simulink model "demo"  (R2019a)
settings: Solver=FixedStepAuto  StartTime=0.0  StopTime=inf  FixedStep=1  RelTol=1e-3
settings Model: Creator=Administrator  LastModifiedBy=Administrator

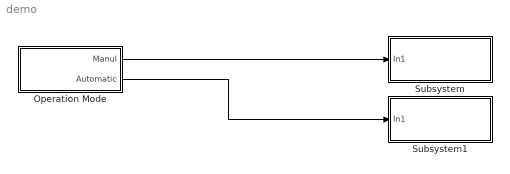
== system demo ==
  Operation Mode : Subsystem
  Subsystem : Subsystem
  Subsystem1 : Subsystem
  wires:
  Operation Mode/2(Automatic) -> Subsystem1/1(In1)
  Operation Mode/1("Manul ") -> Subsystem/1(In1)

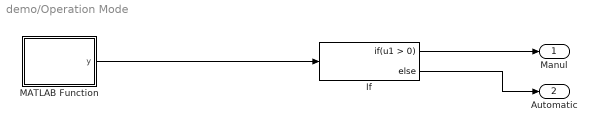
== system demo/Operation Mode ==
  If : If
  MATLAB Function : MATLAB Function  TreatAsAtomicUnit=on
  "Manul " : Outport
  Automatic : Outport  Port=2
  wires:
  If/1 -> "Manul "/1
  If/2 -> Automatic/1
  MATLAB Function/1(y) -> If/1

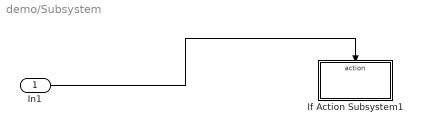
== system demo/Subsystem ==
  In1 : Inport
  If Action Subsystem1 : Subsystem  TreatAsAtomicUnit=on
  wires:
  In1/1 -> If Action Subsystem1/Action

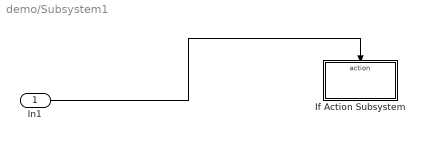
== system demo/Subsystem1 ==
  In1 : Inport
  If Action Subsystem : Subsystem  TreatAsAtomicUnit=on
  wires:
  In1/1 -> If Action Subsystem/Action

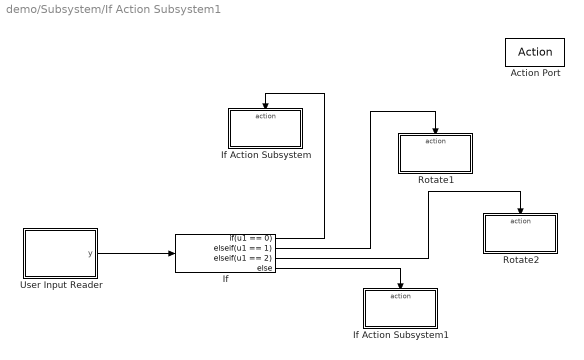
== system demo/Subsystem/If Action Subsystem1 ==
  Action Port : ActionPort
  If : If  IfExpression=u1 == 0  ElseIfExpressions=u1 == 1, u1 == 2
  If Action Subsystem : Subsystem  TreatAsAtomicUnit=on
  If Action Subsystem1 : Subsystem  TreatAsAtomicUnit=on
  Rotate1 : Subsystem  TreatAsAtomicUnit=on
  Rotate2 : Subsystem  TreatAsAtomicUnit=on
  User Input Reader : MATLAB Function  TreatAsAtomicUnit=on
  wires:
  User Input Reader/1(y) -> If/1
  If/2 -> Rotate1/Action
  If/3 -> Rotate2/Action
  If/4 -> If Action Subsystem1/Action
  If/1 -> If Action Subsystem/Action

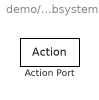
== system demo/Subsystem1/If Action Subsystem ==
  Action Port : ActionPort

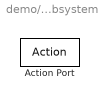
== system demo/Subsystem/If Action Subsystem1/If Action Subsystem ==
  Action Port : ActionPort

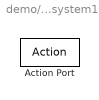
== system demo/Subsystem/If Action Subsystem1/If Action Subsystem1 ==
  Action Port : ActionPort

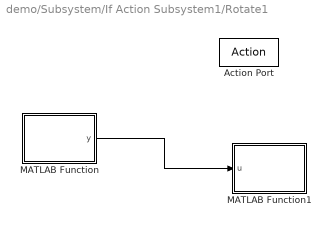
== system demo/Subsystem/If Action Subsystem1/Rotate1 ==
  Action Port : ActionPort
  MATLAB Function : MATLAB Function  TreatAsAtomicUnit=on
  MATLAB Function1 : MATLAB Function  TreatAsAtomicUnit=on
  wires:
  MATLAB Function/1(y) -> MATLAB Function1/1(u)

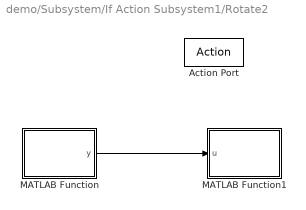
== system demo/Subsystem/If Action Subsystem1/Rotate2 ==
  Action Port : ActionPort
  MATLAB Function : MATLAB Function  TreatAsAtomicUnit=on
  MATLAB Function1 : MATLAB Function  TreatAsAtomicUnit=on
  wires:
  MATLAB Function/1(y) -> MATLAB Function1/1(u)

== matlab function demo/Operation Mode/MATLAB Function ==
  data: y output
function y = fcn()
coder.extrinsic("xlsread");
y = 0;
%coder.extrinsic('y');

y = xlsread("G2M_current.xls", 'A1:A1');

== matlab function demo/Subsystem/If Action Subsystem1/Rotate1/MATLAB Function ==
  data: y output
%function  fcn(u)

%y = u;
function y = fcn()
coder.extrinsic("system");
system('bacwp.exe 701103 4 6 85 8 -1 9 1');
pause(4);
system('bacwp.exe 701103 4 6 85 8 -1 9 0');
y = 0
end

== matlab function demo/Subsystem/If Action Subsystem1/Rotate1/MATLAB Function1 ==
  data: u input
%function y = fcn(u)

%y = u;
function fcn(u)
coder.extrinsic("xlswrite");
xlswrite('G2A_current.xls',u,'Sheet1','A1');
end

== matlab function demo/Subsystem/If Action Subsystem1/Rotate2/MATLAB Function ==
  data: y output
%function y = fcn(u)

%y = u;
function y = fcn()
coder.extrinsic("system");

system('bacwp.exe 701103 4 7 85 8 -1 9 1');
pause(4);
system('bacwp.exe 701103 4 7 85 8 -1 9 0');
y = 0;
end

== matlab function demo/Subsystem/If Action Subsystem1/Rotate2/MATLAB Function1 ==
  data: u input
%function y = fcn(u)

%y = u;
function fcn(u)
coder.extrinsic("xlswrite");
xlswrite('G2A_current.xls',u,'Sheet1','A1');

end

== matlab function demo/Subsystem/If Action Subsystem1/User Input Reader ==
  data: y output
 function y = fcn()
coder.extrinsic("xlsread");
y = 0;
%coder.extrinsic('y');

y = xlsread("G2A_current.xls","A1:A1");
